simulink model "Q1_on_off_controller"  (R2018a)
settings: Solver=FixedStepDiscrete  StartTime=0.0  StopTime=15  FixedStep=50e-6  RelTol=1e-3
libraries: powerlib x5, electricdrivelib x1, simulink_extras x1, dspsigops x1
settings Model: Creator=nailt  LastModifiedBy=nailt

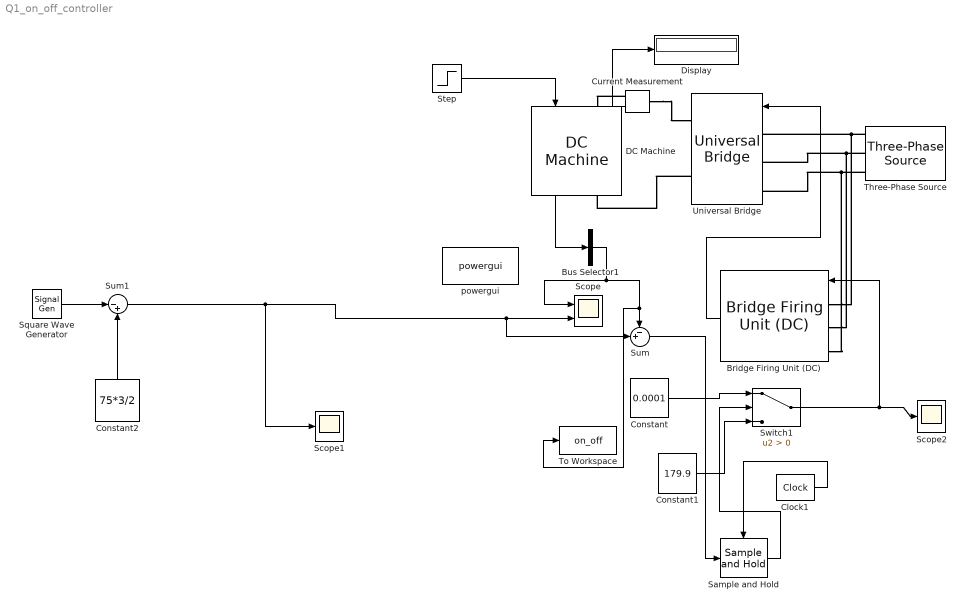
== system Q1_on_off_controller ==
  Bridge Firing Unit (DC) : electricdrivelib/Fundamental Drive Blocks/Bridge Firing Unit (DC)  OverrideUsingVariant=AC_Detailed_two quadrant  detailLevel=Detailed  nbPhases=3  numQuad=2  x4=50  x9=10  Ts=50e-6
      settings: SourceProductName=Simscape Power Systems  SourceProductBaseCode=PS
  Bus Selector1 : BusSelector  OutputSignals=Speed wm (rad/s)  OutputAsBus=on
  Clock1 : simulink_extras/Flip Flops/Clock  period=1/50
  Constant : Constant  Value=0.0001
  Constant1 : Constant  Value=179.9
  Constant2 : Constant  Value=75*3/2
  Current Measurement : powerlib/Measurements/Current Measurement  PhasorSimulation=off  OutputType=Complex  PSBequivalent=0
  DC Machine : powerlib/Machines/DC Machine  PresetModel=No  MechanicalLoad=Torque TL  FieldType=Permanent magnet  ShowDetailedParameters=on  MeasurementBus=off  RLa=[10 0.1]  RLf=[281.3 156]  Laf=0.9483  MachineConstant=Back-emf constant (V/rpm)  Ke=0.3  Kt=1.8  J=0.4  Bm=0.002953  Tf=0.5161  w0=1  Ifinit=1  TsPowergui=0  TsBlock=-1
  Display : Display
  Sample and Hold : dspsigops/Sample and Hold  trig=Rising edge  initCond=0  latchinput=off
  Scope : Scope  NumInputPorts=2
  Scope1 : Scope
  Scope2 : Scope
  Square Wave Generator : SignalGenerator  WaveForm=square  Amplitude=75/2  Frequency=1/9
  Step : Step  Time=0.001  After=24  SampleTime=0
  Sum : Sum  Inputs=-+|
  Sum1 : Sum  Inputs=|-+
  Switch1 : Switch  Criteria=u2 > Threshold
  Three-Phase Source : powerlib/Electrical Sources/Three-Phase Source  InternalConnection=Yg  VoltagePhases=off  Voltage=400  PhaseAngle=0  Voltage_phases=[25e3 25e3 25e3]/sqrt(3)  PhaseAngles_phases=[0 -120 +120]  Frequency=50  NonIdealSource=on  SpecifyImpedance=off  Resistance=100e-3  Inductance=100e-6  ShortCircuitLevel=100e6  BaseVoltage=25e3  XRratio=7  BusType=swing  Pref=10e3  Qref=0  Prefabc=[10e3, 10e3, 10e3]  Qrefabc=[0, 0, 0]  Qmin=-inf  Qmax=inf
  To Workspace : ToWorkspace  VariableName=on_off  SaveFormat=Timeseries  SampleTime=-1
  Universal Bridge : powerlib/Power Electronics/Universal Bridge  Arms=3  SnubberResistance=1e10  SnubberCapacitance=inf  Device=Thyristors  Ron=20e-3  Lon=0  ForwardVoltages="[  0  0  ]"  ForwardVoltage=0.8  GTOparameters=[ 10e-6 , 20e-6 ]  IGBTparameters=[ 1e-6 , 2e-6 ]  Measurements=None  Measurements_2=None  converterType=Rectifier
  powergui : powerlib/powergui  Priority=1  SimulationMode=Discrete  SampleTime=50e-6  frequency=60  Iterations=50  frequencyindice=50  Pbase=100e6  ErrMax=1e-4  UnitsV=kV  UnitsW=MW  buscounter=0  FunctionMessages=off  echomessages=off  EnableUseOfTLC=off  CurrentSourceSwitches=off  DisableSnubberDevices=off  DisableRonSwitches=off  DisableVfSwitches=off  DisplayEquations=off  SolverType=Tustin/Backward Euler (TBE)  Interpol=off  ExternalGateDelay=off  methode=off  Ts=100  x0status=blocks  SPID=on  SwTol=0  HookPort=off  RestoreLinks=warning  ResistiveCurrentMeasurement=off  Frange=[0:2:500]  Ylog=off  Xlog=on  ShowGrid=off  save=off  variable=ZData  structure=0  ZoomFFT=off  StartTime=0.0  cycles=1  DisplayStyle=1  fundamental=60  FreqAxis=off  MaxFrequency=1000  frequencyindicesteady=1  RmsSteady=1  display=off
  wires:
  Step/1 -> DC Machine/1
  Bridge Firing Unit (DC)/1 -> Universal Bridge/1
  Current Measurement/1 -> Display/1
  Constant/1 -> Switch1/1
  Constant1/1 -> Switch1/3
  DC Machine/1 -> Bus Selector1/1
  Bus Selector1/1 -> To Workspace/1, Sum/1, Scope/1
  Clock1/1 -> Sample and Hold/Trigger
  Sum/1 -> Sample and Hold/1
  Sample and Hold/1 -> Switch1/2
  Constant2/1 -> Sum1/2
  Square Wave Generator/1 -> Sum1/1
  Sum1/1 -> Scope1/1, Sum/2, Scope/2
  Switch1/1 -> Scope2/1, Bridge Firing Unit (DC)/1
  connections:
  Three-Phase Source/RConn1 -- Bridge Firing Unit (DC)/LConn1 -- Universal Bridge/LConn1
  Three-Phase Source/RConn2 -- Bridge Firing Unit (DC)/LConn2 -- Universal Bridge/LConn2
  Three-Phase Source/RConn3 -- Bridge Firing Unit (DC)/LConn3 -- Universal Bridge/LConn3
  Universal Bridge/RConn2 -- DC Machine/RConn1
  Current Measurement/LConn1 -- Universal Bridge/RConn1
  Current Measurement/RConn1 -- DC Machine/LConn1
